simulink model "symproblem3"  (R2022a)
settings: Solver=VariableStepAuto  StartTime=0.0  StopTime=10.0  RelTol=1e-3
values from neighbouring files (symbols this model uses):
  Cx = 0.4    [Problem3.m]
  g = 9.81    [Problem3.m]
  m = 2.5    [Problem3.m]
  vw = 3    [Problem3.m]
  vx = v*cos(la)    [Problem3.m]
  vy = v*sin(la)    [Problem3.m]
settings Model: Creator=77dal  LastModifiedBy=77dal

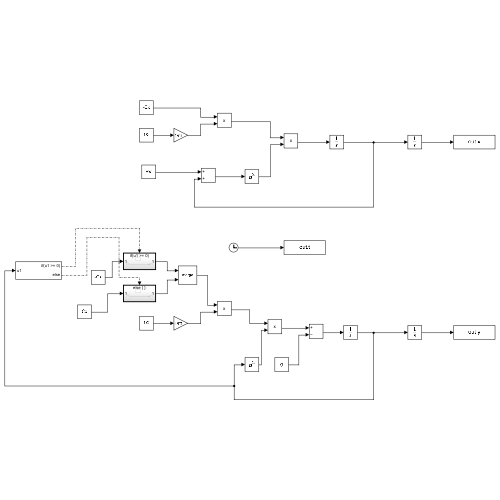
[thumbnail: Simulink's stored preview of the top-level diagram]
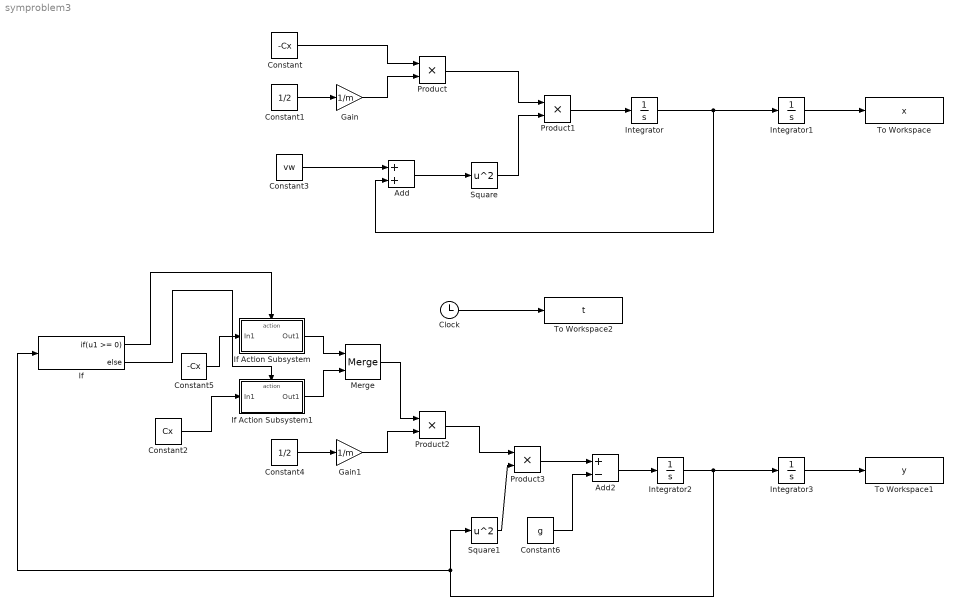
== system symproblem3 ==
  Add : Sum
  Add2 : Sum  Inputs=+-
  Clock : Clock
  Constant : Constant  Value=-Cx
  Constant1 : Constant  Value=1/2
  Constant2 : Constant  Value=Cx
  Constant3 : Constant  Value=vw
  Constant4 : Constant  Value=1/2
  Constant5 : Constant  Value=-Cx
  Constant6 : Constant  Value=g
  Gain : Gain  Gain=1/m
  Gain1 : Gain  Gain=1/m
  If : If  IfExpression=u1 >= 0
  If Action Subsystem : Subsystem  TreatAsAtomicUnit=on
  If Action Subsystem1 : Subsystem  TreatAsAtomicUnit=on
  Integrator : Integrator  InitialCondition=vx
  Integrator1 : Integrator
  Integrator2 : Integrator  InitialCondition=vy
  Integrator3 : Integrator  InitialCondition=1
  Merge : Merge
  Product{,1..3} (4 alike) : Product
  Square : Math  Operator=square
  Square1 : Math  Operator=square
  To Workspace : ToWorkspace  VariableName=x  SampleTime=-1
  To Workspace1 : ToWorkspace  VariableName=y  SampleTime=-1
  To Workspace2 : ToWorkspace  VariableName=t  SampleTime=-1
  wires:
  Constant1/1 -> Gain/1
  Constant/1 -> Product/1
  Gain/1 -> Product/2
  Constant3/1 -> Add/1
  Add/1 -> Square/1
  Product/1 -> Product1/1
  Square/1 -> Product1/2
  Product1/1 -> Integrator/1
  Integrator/1 -> Add/2, Integrator1/1
  Integrator1/1 -> To Workspace/1
  Integrator3/1 -> To Workspace1/1
  Integrator2/1 -> If/1, Square1/1, Integrator3/1
  Product2/1 -> Product3/1
  Square1/1 -> Product3/2
  Gain1/1 -> Product2/2
  Constant4/1 -> Gain1/1
  Constant6/1 -> Add2/2
  Add2/1 -> Integrator2/1
  Product3/1 -> Add2/1
  Clock/1 -> To Workspace2/1
  If/1 -> If Action Subsystem/Action
  If/2 -> If Action Subsystem1/Action
  If Action Subsystem/1(Out1) -> Merge/1
  If Action Subsystem1/1(Out1) -> Merge/2
  Constant2/1 -> If Action Subsystem1/1(In1)
  Constant5/1 -> If Action Subsystem/1(In1)
  Merge/1 -> Product2/1

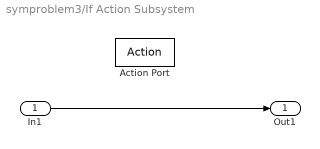
== system symproblem3/If Action Subsystem ==
  In1 : Inport
  Action Port : ActionPort  ActionPortLabel=if(u1 >= 0)
  Out1 : Outport
  wires:
  In1/1 -> Out1/1

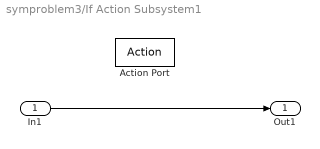
== system symproblem3/If Action Subsystem1 ==
  In1 : Inport
  Action Port : ActionPort  ActionPortLabel=else
  Out1 : Outport
  wires:
  In1/1 -> Out1/1
